simulink model "withFtr"  (R2020a)
settings: Solver=VariableStepAuto  StartTime=0.0  StopTime=30  RelTol=1e-3
values from neighbouring files (symbols this model uses):
  F_1 = 0.03    [Experiments.m]    (also in Pendulum_Final.mat; Pendulum_Final_Estimated.mat; withFtr_final.m)
  F_2 = 0.03    [Experiments.m]    (also in Pendulum_Final.mat; Pendulum_Final_Estimated.mat = 0.0252847335501; withFtr_final.m)
  g = 9.81    [Experiments.m]    (also in Pendulum_Final.mat = 9.875; Pendulum_Final_Estimated.mat; withFtr_final.m)
  I = m*L^2/3    (= 0.0106666666667)    [Experiments.m]    (also in Pendulum_Final.mat; Pendulum_Final_Estimated.mat = 0.0426666666667; withFtr_final.m = 0.0426666666667)
  initials = [0 0 2 0]    [Pendulum_Final.mat]    (also in Pendulum_Final_Estimated.mat = [0 0 4.16014904948 2.64412669288])
  K = [-1 -1.92347126743 -18.2101463629 -4.01241025286]    [Pendulum_Final.mat]    (also in Pendulum_Final_Estimated.mat = [-1 -2.10537488633 -21.7109079068 -6.29681075916])
  L = 0.4    [Experiments.m]    (also in Pendulum_Final.mat; Pendulum_Final_Estimated.mat; withFtr_final.m)
  m = 0.2    [Experiments.m]    (also in Pendulum_Final.mat; Pendulum_Final_Estimated.mat = 0.398406265639; withFtr_final.m)
  M = 0.36    [Experiments.m]    (also in Pendulum_Final.mat; Pendulum_Final_Estimated.mat; withFtr_final.m)
settings Model: Creator=pazh2  LastModifiedBy=pazh2

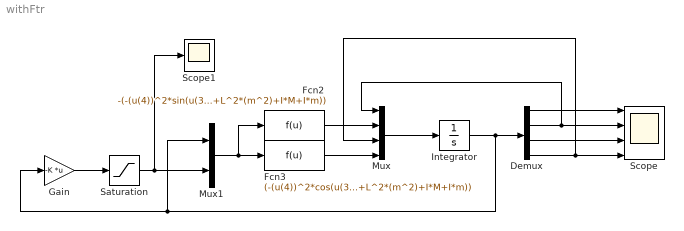
== system withFtr ==
  Demux : Demux
  Fcn2 : Fcn  Expr=-(-(u(4))^2*sin(u(3))*(L^3)*(m^2)+cos(u(3))*sin(u(3))*g*(L^2)*(m^2)-I*((u(4))^2)*sin(u(3))*L*m+F_1*(u(2))*(L^2)*m-F_2*(u(4))*cos(u(3))*L*m-u(5)*(L^2)*m+I*F_1*(u(2))-I*u(5))*(1/(-cos(u(3))^2*(L^2)*(m^2)+M*(L^2)*m+L^2*(m^2)+I*M+I*m))
  Fcn3 : Fcn  Expr=(-(u(4))^2*cos(u(3))*sin(u(3))*(L^2)*(m^2)+F_1*(u(2))*cos(u(3))*L*m+M*sin(u(3))*g*L*m+sin(u(3))*g*L*(m^2)-cos(u(3))*u(5)*L*m-F_2*M*(u(4))-F_2*(u(4))*m)*(1/(-cos(u(3))^2*(L^2)*(m^2)+M*(L^2)*m+L^2*(m^2)+I*M+I*m))
  Gain : Gain  Gain=-K  Multiplication=Matrix(K*u)
  Integrator : Integrator  InitialCondition=initials
  Mux : Mux
  Mux1 : Mux  Inputs=2
  Saturation : Saturate  UpperLimit=14  LowerLimit=-14
  Scope : Scope  NumInputPorts=4
  Scope1 : Scope
  wires:
  Mux/1 -> Integrator/1
  Demux/4 -> Mux/3, Scope/4
  Fcn3/1 -> Mux/4
  Fcn2/1 -> Mux/2
  Demux/1 -> Scope/1
  Demux/3 -> Scope/3
  Demux/2 -> Mux/1, Scope/2
  Mux1/1 -> Fcn2/1, Fcn3/1
  Integrator/1 -> Mux1/1, Gain/1, Demux/1
  Gain/1 -> Saturation/1
  Saturation/1 -> Scope1/1, Mux1/2
